simulink model "bancodepi"  (Simulink 5.0)
settings: Solver=ode45  StartTime=0.0  StopTime=75.0  RelTol=1e-3
undefined symbols (not defined in the file): q, Vd, Vm
libraries: simulink_extras x3
settings Model: LastModifiedBy=pc1

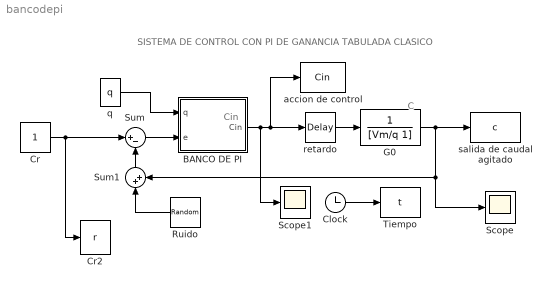
== system bancodepi ==
  note: Cin
  note: C
  note: SISTEMA DE CONTROL CON PI DE GANANCIA TABULADA CLASICO
  BANCO DE PI : Subsystem
  Clock : Clock
      settings: Decimation=10
  Cr : Constant
  Cr2 : ToWorkspace  VariableName=r  SampleTime=-1  SaveFormat=Array
  G0 : TransferFcn  Denominator=[Vm/q 1]
  Ruido : RandomNumber  Orientation=left  Variance=0.01  Seed=5  SampleTime=0.1
  Scope : Scope
  Scope1 : Scope
  Sum : Sum  Inputs=|+-  SaturateOnIntegerOverflow=on
  Sum1 : Sum  Orientation=up  Inputs=|++  SaturateOnIntegerOverflow=on
  Tiempo : ToWorkspace  VariableName=t  SampleTime=-1  SaveFormat=Array
  accion de control : ToWorkspace  VariableName=Cin  SampleTime=-1  SaveFormat=Array
  q : Constant  Value=q
  retardo : TransportDelay  DelayTime=Vd/q
  salida de caudal agitado : ToWorkspace  VariableName=c  SampleTime=-1  SaveFormat=Array
  wires:
  BANCO DE PI/1(Cin) -> retardo/1, accion de control/1, Scope1/1
  retardo/1 -> G0/1
  G0/1 -> salida de caudal agitado/1, Scope/1, Sum1/2
  Clock/1 -> Tiempo/1
  Sum/1 -> BANCO DE PI/2(e)
  Cr/1 -> Sum/1, Cr2/1
  q/1 -> BANCO DE PI/1(q)
  Sum1/1 -> Sum/2
  Ruido/1 -> Sum1/1

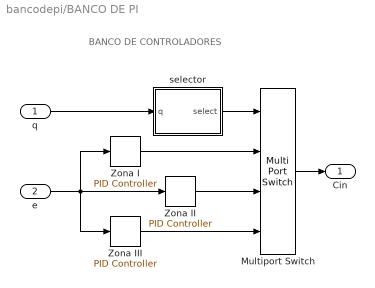
== system bancodepi/BANCO DE PI ==
  note: BANCO DE CONTROLADORES
  q : Inport
  e : Inport  Port=2
  Multiport Switch : MultiPortSwitch  Inputs=3  SaturateOnIntegerOverflow=on
  Zona I : simulink_extras/Additional Linear/PID Controller  P=0.2  I=0.2/1.1  D=0
  Zona II : simulink_extras/Additional Linear/PID Controller  P=0.25  I=0.25/0.7  D=0
  Zona III : simulink_extras/Additional Linear/PID Controller  P=0.4  I=0.4/0.8  D=0
  selector : Subsystem
  Cin : Outport
  wires:
  e/1 -> Zona III/1, Zona I/1, Zona II/1
  Zona I/1 -> Multiport Switch/2
  Zona II/1 -> Multiport Switch/3
  Zona III/1 -> Multiport Switch/4
  Multiport Switch/1 -> Cin/1
  q/1 -> selector/1(q)
  selector/1(select) -> Multiport Switch/1

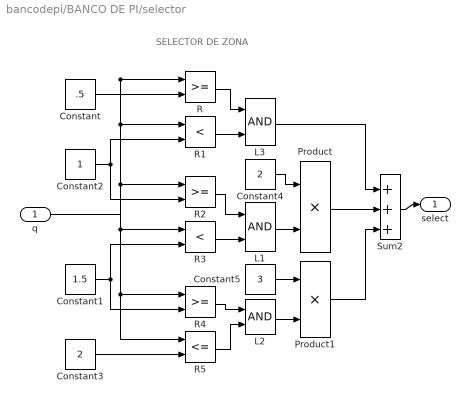
== system bancodepi/BANCO DE PI/selector ==
  note: SELECTOR DE ZONA
  q : Inport
  Constant : Constant  Value=.5
  Constant1 : Constant  Value=1.5
  Constant2 : Constant
  Constant3 : Constant  Value=2
  Constant4 : Constant  Value=2
  Constant5 : Constant  Value=3
  L1 : Logic  AllPortsSameDT=off
  L2 : Logic  AllPortsSameDT=off
  L3 : Logic  AllPortsSameDT=off
  Product : Product  SaturateOnIntegerOverflow=on
  Product1 : Product  SaturateOnIntegerOverflow=on
  R : RelationalOperator
  R1 : RelationalOperator  Operator=<
  R2 : RelationalOperator
  R3 : RelationalOperator  Operator=<
  R4 : RelationalOperator
  R5 : RelationalOperator  Operator=<=
  Sum2 : Sum  Inputs=|+++  SaturateOnIntegerOverflow=on
  select : Outport
  wires:
  Constant/1 -> R/2
  q/1 -> R/1, R1/1, R2/1, R3/1, R4/1, R5/1
  R/1 -> L3/1
  Constant2/1 -> R1/2, R2/2
  R1/1 -> L3/2
  Constant1/1 -> R3/2, R4/2
  R2/1 -> L1/1
  R3/1 -> L1/2
  Constant3/1 -> R5/2
  R5/1 -> L2/2
  Constant4/1 -> Product/1
  L1/1 -> Product/2
  Constant5/1 -> Product1/1
  L2/1 -> Product1/2
  L3/1 -> Sum2/1
  Product/1 -> Sum2/2
  Product1/1 -> Sum2/3
  Sum2/1 -> select/1
  R4/1 -> L2/1
